simulink model "model_9"  (R2021a)
settings: Solver=VariableStepAuto  StartTime=0.0  StopTime=60.0  RelTol=1e-3
libraries: simulink x1
settings Model: Creator=mansi  LastModifiedBy=mansi

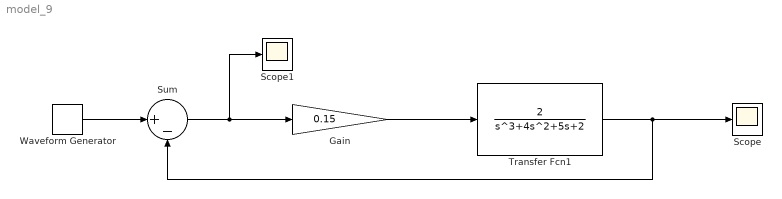
== system model_9 ==
  Gain : Gain  Gain=0.15
  Scope : Scope
  Scope1 : Scope
  Sum : Sum  Inputs=|+-
  Transfer Fcn1 : TransferFcn  Numerator=[2]  Denominator=[1,4,5,2]
  Waveform Generator : simulink/Sources/Waveform Generator  OutMin=[]  OutMax=[]  OutDataTypeStr=double  SelectedSignal=1  Signals=step(0,0,1)  BlockNames=MultiportSwitch_77ad4a2251064ef  SampleTime=0.1
  wires:
  Waveform Generator/1 -> Sum/1
  Transfer Fcn1/1 -> Scope/1, Sum/2
  Sum/1 -> Scope1/1, Gain/1
  Gain/1 -> Transfer Fcn1/1
